simulink model "Discreto"  (R2019a)
settings: Solver=VariableStepAuto  StartTime=0.0  StopTime=30  RelTol=1e-3
settings Model: Creator=STEVEN  LastModifiedBy=STEVEN

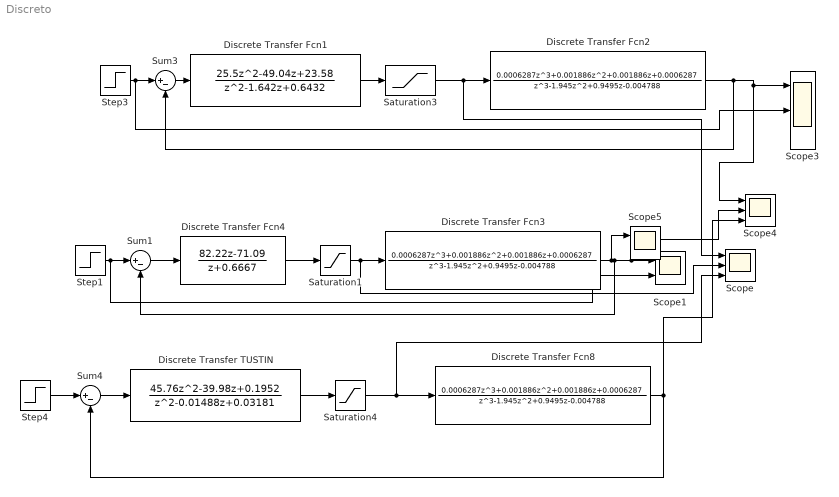
== system Discreto ==
  Discrete Transfer Fcn1 : DiscreteTransferFcn  Numerator=[25.5 -49.04 23.58]  Denominator=[1 -1.642 0.6432]  SampleTime=0.1
  Discrete Transfer Fcn2 : DiscreteTransferFcn  Numerator=[0.0006287 0.001886 0.001886 0.0006287]  Denominator=[1 -1.945 0.9495 -0.004788]  SampleTime=0.1
  Discrete Transfer Fcn3 : DiscreteTransferFcn  Numerator=[0.0006287 0.001886 0.001886 0.0006287]  Denominator=[1 -1.945 0.9495 -0.004788]  SampleTime=0.1
  Discrete Transfer Fcn4 : DiscreteTransferFcn  Numerator=[82.22 -71.09]  Denominator=[1 0.6667]  SampleTime=0.1
  Discrete Transfer Fcn8 : DiscreteTransferFcn  Numerator=[0.0006287 0.001886 0.001886 0.0006287]  Denominator=[1 -1.945 0.9495 -0.004788]  SampleTime=0.1
  Discrete Transfer TUSTIN : DiscreteTransferFcn  Numerator=[45.76 -39.98 0.1952]  Denominator=[1 -0.01488 0.03181]  SampleTime=0.1
  Saturation1 : Saturate  UpperLimit=10  LowerLimit=-10
  Saturation3 : Saturate  UpperLimit=10  LowerLimit=-10
  Saturation4 : Saturate  UpperLimit=10  LowerLimit=-10
  Scope : Scope  NumInputPorts=3
  Scope1 : Scope  NumInputPorts=2
  Scope3 : Scope  NumInputPorts=3
  Scope4 : Scope  NumInputPorts=3
  Scope5 : Scope  NumInputPorts=2
  Step1 : Step  Time=0  SampleTime=0
  Step3 : Step  Time=0  SampleTime=0
  Step4 : Step  Time=0  SampleTime=0
  Sum1 : Sum  Inputs=|+-
  Sum3 : Sum  Inputs=|+-
  Sum4 : Sum  Inputs=|+-
  wires:
  Discrete Transfer Fcn4/1 -> Saturation1/1
  Step1/1 -> Scope1/2, Sum1/1
  Step3/1 -> Scope3/2, Sum3/1
  Sum1/1 -> Discrete Transfer Fcn4/1
  Saturation1/1 -> Discrete Transfer Fcn3/1, Scope/2
  Saturation3/1 -> Discrete Transfer Fcn2/1, Scope/1
  Sum3/1 -> Discrete Transfer Fcn1/1
  Discrete Transfer Fcn1/1 -> Saturation3/1
  Discrete Transfer Fcn2/1 -> Sum3/2, Scope4/1, Scope3/1
  Discrete Transfer Fcn3/1 -> Scope5/1, Scope4/2, Scope1/1, Sum1/2
  Step4/1 -> Sum4/1
  Discrete Transfer TUSTIN/1 -> Saturation4/1
  Saturation4/1 -> Scope/3, Discrete Transfer Fcn8/1
  Sum4/1 -> Discrete Transfer TUSTIN/1
  Discrete Transfer Fcn8/1 -> Scope4/3, Sum4/2
